simulink model "JABS_AutoSave_20200707_1036"  (R2018b)
settings: Solver=FixedStepAuto  StartTime=0.0  StopTime=10.0  FixedStep=0.01  RelTol=1e-3
(part 2 of 2)

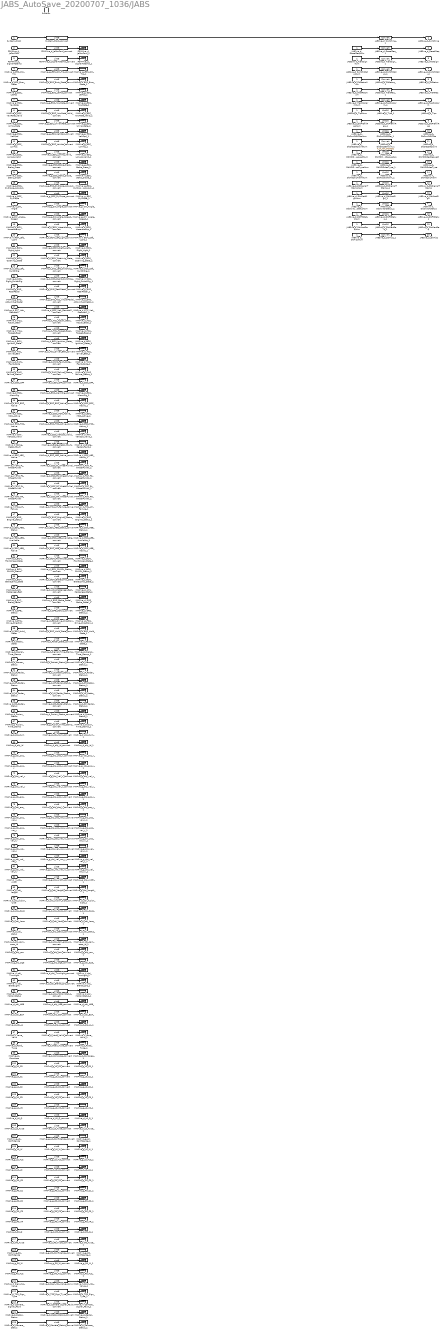
== system JABS_AutoSave_20200707_1036/JABS ==
  System_Clock : Inport  OutDataTypeStr=UInt16
  FDMMve_d_JaFcnConf : Inport  Port=2  OutDataTypeStr=UInt16
  FDMMve_d_SignalTStamp : Inport  Port=3  OutDataTypeStr=UInt16
  IMAPve_g_EPS_SW_Trq : Inport  Port=4  OutDataTypeStr=T_M_Nm_Float32
  IMAPve_d_EPS_Error_State : Inport  Port=5  OutDataTypeStr=UInt16
  IMAPve_g_ESC_LatAcc : Inport  Port=6  OutDataTypeStr=T_M_Nm_Float32
  IMAPve_g_ESC_YawRate : Inport  Port=7  OutDataTypeStr=T_M_Nm_Float32
  IMAPve_d_ESC_YawRate_Valid : Inport  Port=8  OutDataTypeStr=UInt16
  IMAPve_g_ESC_UnYawRate : Inport  Port=9  OutDataTypeStr=T_M_Nm_Float32
  IMAPve_g_ESC_VehSpd : Inport  Port=10  OutDataTypeStr=T_M_Nm_Float32
  IMAPve_g_ESC_LonAcc : Inport  Port=11  OutDataTypeStr=T_M_Nm_Float32
  IMAPve_d_ESC_LonAcc_Valid : Inport  Port=12  OutDataTypeStr=UInt16
  IMAPve_g_ESC_Brake_Press : Inport  Port=13  OutDataTypeStr=T_M_Nm_Float32
  IMAPve_g_ESC_Static_Slope : Inport  Port=14  OutDataTypeStr=T_M_Nm_Float32
  IMAPve_g_ESC_DySlope_Accuracy : Inport  Port=15  OutDataTypeStr=T_M_Nm_Float32
  IMAPve_g_ESC_DySlope : Inport  Port=16  OutDataTypeStr=T_M_Nm_Float32
  IMAPve_g_SW_Angle : Inport  Port=17  OutDataTypeStr=T_M_Nm_Float32
  IMAPve_g_SW_Angle_Speed : Inport  Port=18  OutDataTypeStr=T_M_Nm_Float32
  IMAPve_d_BCM_HazardLamp : Inport  Port=19  OutDataTypeStr=UInt16
  IMAPve_d_BCM_Left_Light : Inport  Port=20  OutDataTypeStr=UInt16
  IMAPve_d_BCM_Right_Light : Inport  Port=21  OutDataTypeStr=UInt16
  IMAPve_d_BCM_Opening_State : Inport  Port=22  OutDataTypeStr=UInt16
  IMAPve_d_SCC_Left_SwitchSig : Inport  Port=23  OutDataTypeStr=UInt16
  IMAPve_d_SCC_Right_SwitchSig : Inport  Port=24  OutDataTypeStr=UInt16
  IMAPve_g_EMS_RealPedal : Inport  Port=25  OutDataTypeStr=T_M_Nm_Float32
  IMAPve_g_EMS_ACC_VirtualPedal : Inport  Port=26  OutDataTypeStr=T_M_Nm_Float32
  IMAPve_d_ESC_Veh_Standstill : Inport  Port=27  OutDataTypeStr=UInt16
  IMAPve_d_TCU_Actual_Gear : Inport  Port=28  OutDataTypeStr=UInt16
  IMAPve_d_TCU_Target_Gear : Inport  Port=29  OutDataTypeStr=UInt16
  IMAPve_d_BCM_Ignition_State : Inport  Port=30  OutDataTypeStr=UInt16
  IMAPve_d_ACU_Driver_Belt : Inport  Port=31  OutDataTypeStr=UInt16
  IMAPve_d_SWS_Fault_Code : Inport  Port=32  OutDataTypeStr=UInt16
  IMAPve_d_SWS_Failure_Status : Inport  Port=33  OutDataTypeStr=UInt16
  IMAPve_d_ESC_OFF : Inport  Port=34  OutDataTypeStr=UInt16
  IMAPve_d_ESC_AlarmSig : Inport  Port=35  OutDataTypeStr=UInt16
  IMAPve_d_ESC_ESC_Active : Inport  Port=36  OutDataTypeStr=UInt16
  IMAPve_d_ESC_MSR_Active : Inport  Port=37  OutDataTypeStr=UInt16
  IMAPve_d_ESC_TCS_Active : Inport  Port=38  OutDataTypeStr=UInt16
  IMAPve_d_ESC_VehSpd_Valid : Inport  Port=39  OutDataTypeStr=UInt16
  IMAPve_d_Brake_Pedal_Fault : Inport  Port=40  OutDataTypeStr=UInt16
  IMAPve_d_ESC_ABS_Active : Inport  Port=41  OutDataTypeStr=UInt16
  IMAPve_d_ESC_FL_WheelPulVal : Inport  Port=42  OutDataTypeStr=UInt16
  IMAPve_d_ESC_FR_WheelPulVal : Inport  Port=43  OutDataTypeStr=UInt16
  IMAPve_d_ESC_RL_WheelPulVal : Inport  Port=44  OutDataTypeStr=UInt16
  IMAPve_d_ESC_RR_WheelPulVal : Inport  Port=45  OutDataTypeStr=UInt16
  IMAPve_d_TCU_AT_Failure : Inport  Port=46  OutDataTypeStr=UInt16
  IMAPve_d_EMS_Engine_Status : Inport  Port=47  OutDataTypeStr=UInt16
  IMAPve_d_ESC_AEB_Status : Inport  Port=48  OutDataTypeStr=UInt16
  IMAPve_d_ESC_AEB_Available : Inport  Port=49  OutDataTypeStr=UInt16
  IMAPve_d_ESC_AEB_Active : Inport  Port=50  OutDataTypeStr=UInt16
  IMAPve_d_BCM_FrontWiper_State : Inport  Port=51  OutDataTypeStr=UInt16
  IMAPve_d_BCM_CHMSL_Status : Inport  Port=52  OutDataTypeStr=UInt16
  IMAPve_d_BCM_BrakeLamp_State : Inport  Port=53  OutDataTypeStr=UInt16
  IMAPve_d_ACU_Passenger_Belt : Inport  Port=54  OutDataTypeStr=UInt16
  IMAPve_d_EMS_Brake_Pedal : Inport  Port=55  OutDataTypeStr=UInt16
  IMAPve_d_EPB_Status : Inport  Port=56  OutDataTypeStr=UInt16
  IMAPve_d_ESC_Drive_Direction : Inport  Port=57  OutDataTypeStr=UInt16
  IMAPve_d_ESC_Hold_State : Inport  Port=58  OutDataTypeStr=UInt16
  IMAPve_d_Radar_State : Inport  Port=59  OutDataTypeStr=UInt16
  IMAPve_d_Signal_Time_Stamp : Inport  Port=60  OutDataTypeStr=UInt16
  IMAPve_d_Sensor_Status : Inport  Port=61  OutDataTypeStr=UInt16
  IMAPve_d_LF_Radar_Status : Inport  Port=62  OutDataTypeStr=UInt16
  IMAPve_d_RF_Radar_Status : Inport  Port=63  OutDataTypeStr=UInt16
  IMAPve_d_LR_Radar_Status : Inport  Port=64  OutDataTypeStr=UInt16
  IMAPve_d_RR_Radar_Status : Inport  Port=65  OutDataTypeStr=UInt16
  IMAPve_d_Fusion_Status : Inport  Port=66  OutDataTypeStr=UInt16
  IMAPve_g_Fusion_Time_Stamp : Inport  Port=67  OutDataTypeStr=T_M_Nm_Float32
  IMAPve_d_obj_Num : Inport  Port=68  OutDataTypeStr=UInt16
  IMAPva_d_obj_id : Inport  Port=69  OutDataTypeStr=UInt16  PortDimensions=40
  IMAPva_g_obj_pos_x : Inport  Port=70  OutDataTypeStr=T_M_Nm_Float32  PortDimensions=40
  IMAPva_g_obj_pos_y : Inport  Port=71  OutDataTypeStr=T_M_Nm_Float32  PortDimensions=40
  IMAPva_g_obj_vel_x : Inport  Port=72  OutDataTypeStr=T_M_Nm_Float32  PortDimensions=40
  IMAPva_g_obj_vel_y : Inport  Port=73  OutDataTypeStr=T_M_Nm_Float32  PortDimensions=40
  IMAPva_g_obj_acc_x : Inport  Port=74  OutDataTypeStr=T_M_Nm_Float32  PortDimensions=40
  IMAPva_g_obj_acc_y : Inport  Port=75  OutDataTypeStr=T_M_Nm_Float32  PortDimensions=40
  IMAPva_g_obj_pos_var_x : Inport  Port=76  OutDataTypeStr=T_M_Nm_Float32  PortDimensions=40
  IMAPva_g_obj_pos_var_y : Inport  Port=77  OutDataTypeStr=T_M_Nm_Float32  PortDimensions=40
  IMAPva_g_obj_pos_var_xy : Inport  Port=78  OutDataTypeStr=T_M_Nm_Float32  PortDimensions=40
  IMAPva_g_obj_vel_var_x : Inport  Port=79  OutDataTypeStr=T_M_Nm_Float32  PortDimensions=40
  IMAPva_g_obj_vel_var_y : Inport  Port=80  OutDataTypeStr=T_M_Nm_Float32  PortDimensions=40
  IMAPva_g_obj_vel_var_xy : Inport  Port=81  OutDataTypeStr=T_M_Nm_Float32  PortDimensions=40
  IMAPva_g_obj_width : Inport  Port=82  OutDataTypeStr=T_M_Nm_Float32  PortDimensions=40
  IMAPva_g_obj_length : Inport  Port=83  OutDataTypeStr=T_M_Nm_Float32  PortDimensions=40
  IMAPva_d_obj_fusion_type : Inport  Port=84  OutDataTypeStr=UInt16  PortDimensions=40
  IMAPva_d_obj_class : Inport  Port=85  OutDataTypeStr=UInt16  PortDimensions=40
  IMAPva_d_obj_lane : Inport  Port=86  OutDataTypeStr=UInt16  PortDimensions=40
  IMAPva_d_obj_status : Inport  Port=87  OutDataTypeStr=UInt16  PortDimensions=40
  IMAPva_d_obj_cam_asso_id : Inport  Port=88  OutDataTypeStr=UInt16  PortDimensions=40
  IMAPva_g_obj_con : Inport  Port=89  OutDataTypeStr=T_M_Nm_Float32  PortDimensions=40
  IMAPva_g_obj_age : Inport  Port=90  OutDataTypeStr=T_M_Nm_Float32  PortDimensions=40
  IMAPva_d_obj_TurnLight : Inport  Port=91  OutDataTypeStr=UInt16  PortDimensions=40
  IMAPva_d_obj_BrakeLight : Inport  Port=92  OutDataTypeStr=UInt16  PortDimensions=40
  IMAPva_d_obj_MotionStatus : Inport  Port=93  OutDataTypeStr=UInt16  PortDimensions=40
  IMAPva_d_obj_AEB : Inport  Port=94  OutDataTypeStr=UInt16  PortDimensions=40
  IMAPva_d_obj_ESA : Inport  Port=95  OutDataTypeStr=UInt16  PortDimensions=40
  IMAPva_d_obj_JA : Inport  Port=96  OutDataTypeStr=UInt16  PortDimensions=40
  IMAPve_d_Lane_Valid : Inport  Port=97  OutDataTypeStr=UInt16
  IMAPve_d_Road_Type : Inport  Port=98  OutDataTypeStr=UInt16
  IMAPve_d_ConsArea : Inport  Port=99  OutDataTypeStr=UInt16
  IMAPve_g_L0_C0 : Inport  Port=100  OutDataTypeStr=T_M_Nm_Float32
  IMAPve_g_L0_C1 : Inport  Port=101  OutDataTypeStr=T_M_Nm_Float32
  IMAPve_g_L0_C2 : Inport  Port=102  OutDataTypeStr=T_M_Nm_Float32
  IMAPve_g_L0_C3 : Inport  Port=103  OutDataTypeStr=T_M_Nm_Float32
  IMAPve_g_L0_VR : Inport  Port=104  OutDataTypeStr=T_M_Nm_Float32
  IMAPve_d_L0_Q : Inport  Port=105  OutDataTypeStr=UInt16
  IMAPve_d_L0_Type : Inport  Port=106  OutDataTypeStr=UInt16
  IMAPve_g_L0_Confidence : Inport  Port=107  OutDataTypeStr=T_M_Nm_Float32
  IMAPve_g_L0_W : Inport  Port=108  OutDataTypeStr=T_M_Nm_Float32
  IMAPve_g_L0_TLC : Inport  Port=109  OutDataTypeStr=T_M_Nm_Float32
  IMAPve_d_L0_LC : Inport  Port=110  OutDataTypeStr=UInt16
  IMAPve_g_R0_C0 : Inport  Port=111  OutDataTypeStr=T_M_Nm_Float32
  IMAPve_g_R0_C1 : Inport  Port=112  OutDataTypeStr=T_M_Nm_Float32
  IMAPve_g_R0_C2 : Inport  Port=113  OutDataTypeStr=T_M_Nm_Float32
  IMAPve_g_R0_C3 : Inport  Port=114  OutDataTypeStr=T_M_Nm_Float32
  IMAPve_g_R0_VR : Inport  Port=115  OutDataTypeStr=T_M_Nm_Float32
  IMAPve_d_R0_Q : Inport  Port=116  OutDataTypeStr=UInt16
  IMAPve_d_R0_Type : Inport  Port=117  OutDataTypeStr=UInt16
  IMAPve_g_R0_Confidence : Inport  Port=118  OutDataTypeStr=T_M_Nm_Float32
  IMAPve_g_R0_W : Inport  Port=119  OutDataTypeStr=T_M_Nm_Float32
  IMAPve_g_R0_TLC : Inport  Port=120  OutDataTypeStr=T_M_Nm_Float32
  IMAPve_d_Sign_ISA_Value : Inport  Port=121  OutDataTypeStr=UInt16
  IMAPve_d_TSR_Sign_Type : Inport  Port=122  OutDataTypeStr=UInt16
  IMAPve_d_Camera_Signal_Fault : Inport  Port=123  OutDataTypeStr=UInt16
  IMAPve_d_Radar_Status : Inport  Port=124  OutDataTypeStr=UInt16
  IMAPve_d_Camera_Status : Inport  Port=125  OutDataTypeStr=UInt16
  function : TriggerPort  TriggerType=function-call  VariantControl=Variant  SampleTimeType=periodic  SampleTime=-1
  FDMMve_d_JaFcnConf_1 : Terminator
  FDMMve_d_JaFcnConf_convert : DataTypeConversion  OutDataTypeStr=uint8
  FDMMve_d_SignalTStamp_1 : Terminator
  FDMMve_d_SignalTStamp_convert : DataTypeConversion  OutDataTypeStr=uint8
  IMAPva_d_obj_AEB_1 : Terminator
  IMAPva_d_obj_AEB_convert : DataTypeConversion  OutDataTypeStr=uint8
  IMAPva_d_obj_BrakeLight_1 : Terminator
  IMAPva_d_obj_BrakeLight_convert : DataTypeConversion  OutDataTypeStr=uint8
  IMAPva_d_obj_ESA_1 : Terminator
  IMAPva_d_obj_ESA_convert : DataTypeConversion  OutDataTypeStr=uint8
  IMAPva_d_obj_JA_1 : Terminator
  IMAPva_d_obj_JA_convert : DataTypeConversion  OutDataTypeStr=uint8
  IMAPva_d_obj_MotionStatus_1 : Terminator
  IMAPva_d_obj_MotionStatus_convert : DataTypeConversion  OutDataTypeStr=uint8
  IMAPva_d_obj_TurnLight_1 : Terminator
  IMAPva_d_obj_TurnLight_convert : DataTypeConversion  OutDataTypeStr=uint8
  IMAPva_d_obj_cam_asso_id_1 : Terminator
  IMAPva_d_obj_cam_asso_id_convert : DataTypeConversion  OutDataTypeStr=uint8
  IMAPva_d_obj_class_1 : Terminator
  IMAPva_d_obj_class_convert : DataTypeConversion  OutDataTypeStr=uint8
  IMAPva_d_obj_fusion_type_1 : Terminator
  IMAPva_d_obj_fusion_type_convert : DataTypeConversion  OutDataTypeStr=uint8
  IMAPva_d_obj_id_1 : Terminator
  IMAPva_d_obj_id_convert : DataTypeConversion  OutDataTypeStr=uint8
  IMAPva_d_obj_lane_1 : Terminator
  IMAPva_d_obj_lane_convert : DataTypeConversion  OutDataTypeStr=uint8
  IMAPva_d_obj_status_1 : Terminator
  IMAPva_d_obj_status_convert : DataTypeConversion  OutDataTypeStr=uint8
  IMAPva_g_obj_acc_x_1 : Terminator
  IMAPva_g_obj_acc_x_convert : DataTypeConversion  OutDataTypeStr=uint8
  IMAPva_g_obj_acc_y_1 : Terminator
  IMAPva_g_obj_acc_y_convert : DataTypeConversion  OutDataTypeStr=uint8
  IMAPva_g_obj_age_1 : Terminator
  IMAPva_g_obj_age_convert : DataTypeConversion  OutDataTypeStr=uint8
  IMAPva_g_obj_con_1 : Terminator
  IMAPva_g_obj_con_convert : DataTypeConversion  OutDataTypeStr=uint8
  IMAPva_g_obj_length_1 : Terminator
  IMAPva_g_obj_length_convert : DataTypeConversion  OutDataTypeStr=uint8
  IMAPva_g_obj_pos_var_x_1 : Terminator
  IMAPva_g_obj_pos_var_x_convert : DataTypeConversion  OutDataTypeStr=uint8
  IMAPva_g_obj_pos_var_xy_1 : Terminator
  IMAPva_g_obj_pos_var_xy_convert : DataTypeConversion  OutDataTypeStr=uint8
  IMAPva_g_obj_pos_var_y_1 : Terminator
  IMAPva_g_obj_pos_var_y_convert : DataTypeConversion  OutDataTypeStr=uint8
  IMAPva_g_obj_pos_x_1 : Terminator
  IMAPva_g_obj_pos_x_convert : DataTypeConversion  OutDataTypeStr=uint8
  IMAPva_g_obj_pos_y_1 : Terminator
  IMAPva_g_obj_pos_y_convert : DataTypeConversion  OutDataTypeStr=uint8
  IMAPva_g_obj_vel_var_x_1 : Terminator
  IMAPva_g_obj_vel_var_x_convert : DataTypeConversion  OutDataTypeStr=uint8
  IMAPva_g_obj_vel_var_xy_1 : Terminator
  IMAPva_g_obj_vel_var_xy_convert : DataTypeConversion  OutDataTypeStr=uint8
  IMAPva_g_obj_vel_var_y_1 : Terminator
  IMAPva_g_obj_vel_var_y_convert : DataTypeConversion  OutDataTypeStr=uint8
  IMAPva_g_obj_vel_x_1 : Terminator
  IMAPva_g_obj_vel_x_convert : DataTypeConversion  OutDataTypeStr=uint8
  IMAPva_g_obj_vel_y_1 : Terminator
  IMAPva_g_obj_vel_y_convert : DataTypeConversion  OutDataTypeStr=uint8
  IMAPva_g_obj_width_1 : Terminator
  IMAPva_g_obj_width_convert : DataTypeConversion  OutDataTypeStr=uint8
  IMAPve_d_ACU_Driver_Belt_1 : Terminator
  IMAPve_d_ACU_Driver_Belt_convert : DataTypeConversion  OutDataTypeStr=uint8
  IMAPve_d_ACU_Passenger_Belt_1 : Terminator
  IMAPve_d_ACU_Passenger_Belt_convert : DataTypeConversion  OutDataTypeStr=uint8
  IMAPve_d_BCM_BrakeLamp_State_1 : Terminator
  IMAPve_d_BCM_BrakeLamp_State_convert : DataTypeConversion  OutDataTypeStr=uint8
  IMAPve_d_BCM_CHMSL_Status_1 : Terminator
  IMAPve_d_BCM_CHMSL_Status_convert : DataTypeConversion  OutDataTypeStr=uint8
  IMAPve_d_BCM_FrontWiper_State_1 : Terminator
  IMAPve_d_BCM_FrontWiper_State_convert : DataTypeConversion  OutDataTypeStr=uint8
  IMAPve_d_BCM_HazardLamp_1 : Terminator
  IMAPve_d_BCM_HazardLamp_convert : DataTypeConversion  OutDataTypeStr=uint8
  IMAPve_d_BCM_Ignition_State_1 : Terminator
  IMAPve_d_BCM_Ignition_State_convert : DataTypeConversion  OutDataTypeStr=uint8
  IMAPve_d_BCM_Left_Light_1 : Terminator
  IMAPve_d_BCM_Left_Light_convert : DataTypeConversion  OutDataTypeStr=uint8
  IMAPve_d_BCM_Opening_State_1 : Terminator
  IMAPve_d_BCM_Opening_State_convert : DataTypeConversion  OutDataTypeStr=uint8
  IMAPve_d_BCM_Right_Light_1 : Terminator
  IMAPve_d_BCM_Right_Light_convert : DataTypeConversion  OutDataTypeStr=uint8
  IMAPve_d_Brake_Pedal_Fault_1 : Terminator
  IMAPve_d_Brake_Pedal_Fault_convert : DataTypeConversion  OutDataTypeStr=uint8
  IMAPve_d_Camera_Signal_Fault_1 : Terminator
  IMAPve_d_Camera_Signal_Fault_convert : DataTypeConversion  OutDataTypeStr=uint8
  IMAPve_d_Camera_Status_1 : Terminator
  IMAPve_d_Camera_Status_convert : DataTypeConversion  OutDataTypeStr=uint8
  IMAPve_d_ConsArea_1 : Terminator
  IMAPve_d_ConsArea_convert : DataTypeConversion  OutDataTypeStr=uint8
  IMAPve_d_EMS_Brake_Pedal_1 : Terminator
  IMAPve_d_EMS_Brake_Pedal_convert : DataTypeConversion  OutDataTypeStr=uint8
  IMAPve_d_EMS_Engine_Status_1 : Terminator
  IMAPve_d_EMS_Engine_Status_convert : DataTypeConversion  OutDataTypeStr=uint8
  IMAPve_d_EPB_Status_1 : Terminator
  IMAPve_d_EPB_Status_convert : DataTypeConversion  OutDataTypeStr=uint8
  IMAPve_d_EPS_Error_State_1 : Terminator
  IMAPve_d_EPS_Error_State_convert : DataTypeConversion  OutDataTypeStr=uint8
  IMAPve_d_ESC_ABS_Active_1 : Terminator
  IMAPve_d_ESC_ABS_Active_convert : DataTypeConversion  OutDataTypeStr=uint8
  IMAPve_d_ESC_AEB_Active_1 : Terminator
  IMAPve_d_ESC_AEB_Active_convert : DataTypeConversion  OutDataTypeStr=uint8
  IMAPve_d_ESC_AEB_Available_1 : Terminator
  IMAPve_d_ESC_AEB_Available_convert : DataTypeConversion  OutDataTypeStr=uint8
  IMAPve_d_ESC_AEB_Status_1 : Terminator
  IMAPve_d_ESC_AEB_Status_convert : DataTypeConversion  OutDataTypeStr=uint8
  IMAPve_d_ESC_AlarmSig_1 : Terminator
  IMAPve_d_ESC_AlarmSig_convert : DataTypeConversion  OutDataTypeStr=uint8
  IMAPve_d_ESC_Drive_Direction_1 : Terminator
  IMAPve_d_ESC_Drive_Direction_convert : DataTypeConversion  OutDataTypeStr=uint8
  IMAPve_d_ESC_ESC_Active_1 : Terminator
  IMAPve_d_ESC_ESC_Active_convert : DataTypeConversion  OutDataTypeStr=uint8
  IMAPve_d_ESC_FL_WheelPulVal_1 : Terminator
  IMAPve_d_ESC_FL_WheelPulVal_convert : DataTypeConversion  OutDataTypeStr=uint8
  IMAPve_d_ESC_FR_WheelPulVal_1 : Terminator
  IMAPve_d_ESC_FR_WheelPulVal_convert : DataTypeConversion  OutDataTypeStr=uint8
  IMAPve_d_ESC_Hold_State_1 : Terminator
  IMAPve_d_ESC_Hold_State_convert : DataTypeConversion  OutDataTypeStr=uint8
  IMAPve_d_ESC_LonAcc_Valid_1 : Terminator
  IMAPve_d_ESC_LonAcc_Valid_convert : DataTypeConversion  OutDataTypeStr=uint8
  IMAPve_d_ESC_MSR_Active_1 : Terminator
  IMAPve_d_ESC_MSR_Active_convert : DataTypeConversion  OutDataTypeStr=uint8
  IMAPve_d_ESC_OFF_1 : Terminator
  IMAPve_d_ESC_OFF_convert : DataTypeConversion  OutDataTypeStr=uint8
  IMAPve_d_ESC_RL_WheelPulVal_1 : Terminator
  IMAPve_d_ESC_RL_WheelPulVal_convert : DataTypeConversion  OutDataTypeStr=uint8
  IMAPve_d_ESC_RR_WheelPulVal_1 : Terminator
  IMAPve_d_ESC_RR_WheelPulVal_convert : DataTypeConversion  OutDataTypeStr=uint8
  IMAPve_d_ESC_TCS_Active_1 : Terminator
  IMAPve_d_ESC_TCS_Active_convert : DataTypeConversion  OutDataTypeStr=uint8
  IMAPve_d_ESC_VehSpd_Valid_1 : Terminator
  IMAPve_d_ESC_VehSpd_Valid_convert : DataTypeConversion  OutDataTypeStr=uint8
  IMAPve_d_ESC_Veh_Standstill_1 : Terminator
  IMAPve_d_ESC_Veh_Standstill_convert : DataTypeConversion  OutDataTypeStr=uint8
  IMAPve_d_ESC_YawRate_Valid_1 : Terminator
  IMAPve_d_ESC_YawRate_Valid_convert : DataTypeConversion  OutDataTypeStr=uint8
  IMAPve_d_Fusion_Status_1 : Terminator
  IMAPve_d_Fusion_Status_convert : DataTypeConversion  OutDataTypeStr=uint8
  IMAPve_d_L0_LC_1 : Terminator
  IMAPve_d_L0_LC_convert : DataTypeConversion  OutDataTypeStr=uint8
  IMAPve_d_L0_Q_1 : Terminator
  IMAPve_d_L0_Q_convert : DataTypeConversion  OutDataTypeStr=uint8
  IMAPve_d_L0_Type_1 : Terminator
  IMAPve_d_L0_Type_convert : DataTypeConversion  OutDataTypeStr=uint8
  IMAPve_d_LF_Radar_Status_1 : Terminator
  IMAPve_d_LF_Radar_Status_convert : DataTypeConversion  OutDataTypeStr=uint8
  IMAPve_d_LR_Radar_Status_1 : Terminator
  IMAPve_d_LR_Radar_Status_convert : DataTypeConversion  OutDataTypeStr=uint8
  IMAPve_d_Lane_Valid_1 : Terminator
  IMAPve_d_Lane_Valid_convert : DataTypeConversion  OutDataTypeStr=uint8
  IMAPve_d_R0_Q_1 : Terminator
  IMAPve_d_R0_Q_convert : DataTypeConversion  OutDataTypeStr=uint8
  IMAPve_d_R0_Type_1 : Terminator
  IMAPve_d_R0_Type_convert : DataTypeConversion  OutDataTypeStr=uint8
  IMAPve_d_RF_Radar_Status_1 : Terminator
  IMAPve_d_RF_Radar_Status_convert : DataTypeConversion  OutDataTypeStr=uint8
  IMAPve_d_RR_Radar_Status_1 : Terminator
  IMAPve_d_RR_Radar_Status_convert : DataTypeConversion  OutDataTypeStr=uint8
  IMAPve_d_Radar_State_1 : Terminator
  IMAPve_d_Radar_State_convert : DataTypeConversion  OutDataTypeStr=uint8
  IMAPve_d_Radar_Status_1 : Terminator
  IMAPve_d_Radar_Status_convert : DataTypeConversion  OutDataTypeStr=uint8
  IMAPve_d_Road_Type_1 : Terminator
  IMAPve_d_Road_Type_convert : DataTypeConversion  OutDataTypeStr=uint8
  IMAPve_d_SCC_Left_SwitchSig_1 : Terminator
  IMAPve_d_SCC_Left_SwitchSig_convert : DataTypeConversion  OutDataTypeStr=uint8
  IMAPve_d_SCC_Right_SwitchSig_1 : Terminator
  IMAPve_d_SCC_Right_SwitchSig_convert : DataTypeConversion  OutDataTypeStr=uint8
  IMAPve_d_SWS_Failure_Status_1 : Terminator
  IMAPve_d_SWS_Failure_Status_convert : DataTypeConversion  OutDataTypeStr=uint8
  IMAPve_d_SWS_Fault_Code_1 : Terminator
  IMAPve_d_SWS_Fault_Code_convert : DataTypeConversion  OutDataTypeStr=uint8
  IMAPve_d_Sensor_Status_1 : Terminator
  IMAPve_d_Sensor_Status_convert : DataTypeConversion  OutDataTypeStr=uint8
  IMAPve_d_Sign_ISA_Value_1 : Terminator
  IMAPve_d_Sign_ISA_Value_convert : DataTypeConversion  OutDataTypeStr=uint8
  IMAPve_d_Signal_Time_Stamp_1 : Terminator
  IMAPve_d_Signal_Time_Stamp_convert : DataTypeConversion  OutDataTypeStr=uint8
  IMAPve_d_TCU_AT_Failure_1 : Terminator
  IMAPve_d_TCU_AT_Failure_convert : DataTypeConversion  OutDataTypeStr=uint8
  IMAPve_d_TCU_Actual_Gear_1 : Terminator
  IMAPve_d_TCU_Actual_Gear_convert : DataTypeConversion  OutDataTypeStr=uint8
  IMAPve_d_TCU_Target_Gear_1 : Terminator
  IMAPve_d_TCU_Target_Gear_convert : DataTypeConversion  OutDataTypeStr=uint8
  IMAPve_d_TSR_Sign_Type_1 : Terminator
  IMAPve_d_TSR_Sign_Type_convert : DataTypeConversion  OutDataTypeStr=uint8
  IMAPve_d_obj_Num_1 : Terminator
  IMAPve_d_obj_Num_convert : DataTypeConversion  OutDataTypeStr=uint8
  IMAPve_g_EMS_ACC_VirtualPedal_1 : Terminator
  IMAPve_g_EMS_ACC_VirtualPedal_convert : DataTypeConversion  OutDataTypeStr=uint8
  IMAPve_g_EMS_RealPedal_1 : Terminator
  IMAPve_g_EMS_RealPedal_convert : DataTypeConversion  OutDataTypeStr=uint8
  IMAPve_g_EPS_SW_Trq_1 : Terminator
  IMAPve_g_EPS_SW_Trq_convert : DataTypeConversion  OutDataTypeStr=uint8
  IMAPve_g_ESC_Brake_Press_1 : Terminator
  IMAPve_g_ESC_Brake_Press_convert : DataTypeConversion  OutDataTypeStr=uint8
  IMAPve_g_ESC_DySlope_1 : Terminator
  IMAPve_g_ESC_DySlope_Accuracy_1 : Terminator
  IMAPve_g_ESC_DySlope_Accuracy_convert : DataTypeConversion  OutDataTypeStr=uint8
  IMAPve_g_ESC_DySlope_convert : DataTypeConversion  OutDataTypeStr=uint8
  IMAPve_g_ESC_LatAcc_1 : Terminator
  IMAPve_g_ESC_LatAcc_convert : DataTypeConversion  OutDataTypeStr=uint8
  IMAPve_g_ESC_LonAcc_1 : Terminator
  IMAPve_g_ESC_LonAcc_convert : DataTypeConversion  OutDataTypeStr=uint8
  IMAPve_g_ESC_Static_Slope_1 : Terminator
  IMAPve_g_ESC_Static_Slope_convert : DataTypeConversion  OutDataTypeStr=uint8
  IMAPve_g_ESC_UnYawRate_1 : Terminator
  IMAPve_g_ESC_UnYawRate_convert : DataTypeConversion  OutDataTypeStr=uint8
  IMAPve_g_ESC_VehSpd_1 : Terminator
  IMAPve_g_ESC_VehSpd_convert : DataTypeConversion  OutDataTypeStr=uint8
  IMAPve_g_ESC_YawRate_1 : Terminator
  IMAPve_g_ESC_YawRate_convert : DataTypeConversion  OutDataTypeStr=uint8
  IMAPve_g_Fusion_Time_Stamp_1 : Terminator
  IMAPve_g_Fusion_Time_Stamp_convert : DataTypeConversion  OutDataTypeStr=uint8
  IMAPve_g_L0_C0_1 : Terminator
  IMAPve_g_L0_C0_convert : DataTypeConversion  OutDataTypeStr=uint8
  IMAPve_g_L0_C1_1 : Terminator
  IMAPve_g_L0_C1_convert : DataTypeConversion  OutDataTypeStr=uint8
  IMAPve_g_L0_C2_1 : Terminator
  IMAPve_g_L0_C2_convert : DataTypeConversion  OutDataTypeStr=uint8
  IMAPve_g_L0_C3_1 : Terminator
  IMAPve_g_L0_C3_convert : DataTypeConversion  OutDataTypeStr=uint8
  IMAPve_g_L0_Confidence_1 : Terminator
  IMAPve_g_L0_Confidence_convert : DataTypeConversion  OutDataTypeStr=uint8
  IMAPve_g_L0_TLC_1 : Terminator
  IMAPve_g_L0_TLC_convert : DataTypeConversion  OutDataTypeStr=uint8
  IMAPve_g_L0_VR_1 : Terminator
  IMAPve_g_L0_VR_convert : DataTypeConversion  OutDataTypeStr=uint8
  IMAPve_g_L0_W_1 : Terminator
  IMAPve_g_L0_W_convert : DataTypeConversion  OutDataTypeStr=uint8
  IMAPve_g_R0_C0_1 : Terminator
  IMAPve_g_R0_C0_convert : DataTypeConversion  OutDataTypeStr=uint8
  IMAPve_g_R0_C1_1 : Terminator
  IMAPve_g_R0_C1_convert : DataTypeConversion  OutDataTypeStr=uint8
  IMAPve_g_R0_C2_1 : Terminator
  IMAPve_g_R0_C2_convert : DataTypeConversion  OutDataTypeStr=uint8
  IMAPve_g_R0_C3_1 : Terminator
  IMAPve_g_R0_C3_convert : DataTypeConversion  OutDataTypeStr=uint8
  IMAPve_g_R0_Confidence_1 : Terminator
  IMAPve_g_R0_Confidence_convert : DataTypeConversion  OutDataTypeStr=uint8
  IMAPve_g_R0_TLC_1 : Terminator
  IMAPve_g_R0_TLC_convert : DataTypeConversion  OutDataTypeStr=uint8
  IMAPve_g_R0_VR_1 : Terminator
  IMAPve_g_R0_VR_convert : DataTypeConversion  OutDataTypeStr=uint8
  IMAPve_g_R0_W_1 : Terminator
  IMAPve_g_R0_W_convert : DataTypeConversion  OutDataTypeStr=uint8
  IMAPve_g_SW_Angle_1 : Terminator
  IMAPve_g_SW_Angle_Speed_1 : Terminator
  IMAPve_g_SW_Angle_Speed_convert : DataTypeConversion  OutDataTypeStr=uint8
  IMAPve_g_SW_Angle_convert : DataTypeConversion  OutDataTypeStr=uint8
  JABSve_d_AlertReqNum : Constant  OutDataTypeStr=uint8
  JABSve_d_AlertReq_1 : DataTypeConversion
  JABSve_d_AlertSignNum : Constant  OutDataTypeStr=uint8  SampleTime=-1
  JABSve_d_AlertSign_1 : DataTypeConversion
  JABSve_d_DbAlertReqNum : Constant  OutDataTypeStr=uint8
  JABSve_d_DbAlertReq_1 : DataTypeConversion  OutDataTypeStr=UInt16
  JABSve_d_DbAlertSignNum : Constant  OutDataTypeStr=uint8
  JABSve_d_DbAlertSign_1 : DataTypeConversion  OutDataTypeStr=UInt16
  JABSve_d_DbDecSetpointNum : Constant  OutDataTypeStr=uint8
  JABSve_d_DbDecSetpoint_1 : DataTypeConversion  OutDataTypeStr=T_M_Nm_Float32
  JABSve_d_DbFltStatusNum : Constant  OutDataTypeStr=uint8
  JABSve_d_DbFltStatus_1 : DataTypeConversion  OutDataTypeStr=UInt16
  JABSve_d_DbFunFARCStaNum : Constant  OutDataTypeStr=uint8
  JABSve_d_DbFunFARCSta_1 : DataTypeConversion  OutDataTypeStr=UInt16
  JABSve_d_DbHapticAlarmNum : Constant  OutDataTypeStr=uint8
  JABSve_d_DbHapticAlarm_1 : DataTypeConversion  OutDataTypeStr=UInt16
  JABSve_d_DbMDDdecRequestNum : Constant  OutDataTypeStr=uint8
  JABSve_d_DbMDDdecRequest_1 : DataTypeConversion  OutDataTypeStr=UInt16
  JABSve_d_DbMDDdecTypeNum : Constant  OutDataTypeStr=uint8
  JABSve_d_DbMDDdecType_1 : DataTypeConversion  OutDataTypeStr=UInt16
  JABSve_d_DbPrefillReqNum : Constant  OutDataTypeStr=uint8
  JABSve_d_DbPrefillReq_1 : DataTypeConversion  OutDataTypeStr=UInt16
  JABSve_d_DbSignalTStampNum : Constant  OutDataTypeStr=uint8
  JABSve_d_DbSignalTStamp_1 : DataTypeConversion  OutDataTypeStr=UInt16
  JABSve_d_DbSwitchStatusNum : Constant  OutDataTypeStr=uint8
  JABSve_d_DbSwitchStatus_1 : DataTypeConversion  OutDataTypeStr=UInt16
  JABSve_d_DbTipsNum : Constant  OutDataTypeStr=uint8
  JABSve_d_DbTips_1 : DataTypeConversion
  JABSve_d_DecelReqNum : Constant  OutDataTypeStr=uint8
  JABSve_d_DecelReq_1 : DataTypeConversion
  JABSve_d_FltStatusNum : Constant  OutDataTypeStr=uint8
  JABSve_d_FltStatus_1 : DataTypeConversion
  JABSve_d_HapticAlarmNum : Constant  OutDataTypeStr=uint8
  JABSve_d_HapticAlarm_1 : DataTypeConversion
  JABSve_d_SwitchStatusNum : Constant  OutDataTypeStr=uint8  SampleTime=-1
  JABSve_d_SwitchStatus_1 : DataTypeConversion
  JABSve_d_Switching_1 : DataTypeConversion
  JABSve_d_TipsNum : Constant  OutDataTypeStr=uint8
  JABSve_d_Tips_1 : DataTypeConversion  OutDataTypeStr=UInt16
  System_Clock_convert : DataTypeConversion  OutDataTypeStr=uint8
  JABSve_d_Switching : Outport  OutDataTypeStr=UInt16
  JABSve_d_DecelReq : Outport  Port=2  OutDataTypeStr=T_M_Nm_Float32
  JABSve_d_AlertSign : Outport  Port=3  OutDataTypeStr=UInt16
  JABSve_d_SwitchStatus : Outport  Port=4  OutDataTypeStr=UInt16
  JABSve_d_FltStatus : Outport  Port=5  OutDataTypeStr=UInt16
  JABSve_d_AlertReq : Outport  Port=6  OutDataTypeStr=UInt16
  JABSve_d_HapticAlarm : Outport  Port=7  OutDataTypeStr=UInt16
  JABSve_d_Tips : Outport  Port=8  OutDataTypeStr=UInt16
  JABSve_d_DbPrefillReq : Outport  Port=9  OutDataTypeStr=UInt16
  JABSve_d_DbFunFARCSta : Outport  Port=10  OutDataTypeStr=UInt16
  JABSve_d_DbDecSetpoint : Outport  Port=11  OutDataTypeStr=T_M_Nm_Float32
  JABSve_d_DbMDDdecRequest : Outport  Port=12  OutDataTypeStr=UInt16
  JABSve_d_DbMDDdecType : Outport  Port=13  OutDataTypeStr=UInt16
  JABSve_d_DbHapticAlarm : Outport  Port=14  OutDataTypeStr=UInt16
  JABSve_d_DbSignalTStamp : Outport  Port=15  OutDataTypeStr=UInt16
  JABSve_d_DbAlertSign : Outport  Port=16  OutDataTypeStr=UInt16
  JABSve_d_DbSwitchStatus : Outport  Port=17  OutDataTypeStr=UInt16
  JABSve_d_DbFltStatus : Outport  Port=18  OutDataTypeStr=UInt16
  JABSve_d_DbAlertReq : Outport  Port=19  OutDataTypeStr=UInt16
  JABSve_d_DbTips : Outport  Port=20  OutDataTypeStr=UInt16
  wires:
  System_Clock/1 -> System_Clock_convert/1
  FDMMve_d_JaFcnConf/1 -> FDMMve_d_JaFcnConf_convert/1
  FDMMve_d_JaFcnConf_convert/1 -> FDMMve_d_JaFcnConf_1/1
  FDMMve_d_SignalTStamp/1 -> FDMMve_d_SignalTStamp_convert/1
  FDMMve_d_SignalTStamp_convert/1 -> FDMMve_d_SignalTStamp_1/1
  IMAPve_g_EPS_SW_Trq/1 -> IMAPve_g_EPS_SW_Trq_convert/1
  IMAPve_g_EPS_SW_Trq_convert/1 -> IMAPve_g_EPS_SW_Trq_1/1
  IMAPve_d_EPS_Error_State/1 -> IMAPve_d_EPS_Error_State_convert/1
  IMAPve_d_EPS_Error_State_convert/1 -> IMAPve_d_EPS_Error_State_1/1
  IMAPve_g_ESC_LatAcc/1 -> IMAPve_g_ESC_LatAcc_convert/1
  IMAPve_g_ESC_LatAcc_convert/1 -> IMAPve_g_ESC_LatAcc_1/1
  IMAPve_g_ESC_YawRate/1 -> IMAPve_g_ESC_YawRate_convert/1
  IMAPve_g_ESC_YawRate_convert/1 -> IMAPve_g_ESC_YawRate_1/1
  IMAPve_d_ESC_YawRate_Valid/1 -> IMAPve_d_ESC_YawRate_Valid_convert/1
  IMAPve_d_ESC_YawRate_Valid_convert/1 -> IMAPve_d_ESC_YawRate_Valid_1/1
  IMAPve_g_ESC_UnYawRate/1 -> IMAPve_g_ESC_UnYawRate_convert/1
  IMAPve_g_ESC_UnYawRate_convert/1 -> IMAPve_g_ESC_UnYawRate_1/1
  IMAPve_g_ESC_VehSpd/1 -> IMAPve_g_ESC_VehSpd_convert/1
  IMAPve_g_ESC_VehSpd_convert/1 -> IMAPve_g_ESC_VehSpd_1/1
  IMAPve_g_ESC_LonAcc/1 -> IMAPve_g_ESC_LonAcc_convert/1
  IMAPve_g_ESC_LonAcc_convert/1 -> IMAPve_g_ESC_LonAcc_1/1
  IMAPve_d_ESC_LonAcc_Valid/1 -> IMAPve_d_ESC_LonAcc_Valid_convert/1
  IMAPve_d_ESC_LonAcc_Valid_convert/1 -> IMAPve_d_ESC_LonAcc_Valid_1/1
  IMAPve_g_ESC_Brake_Press/1 -> IMAPve_g_ESC_Brake_Press_convert/1
  IMAPve_g_ESC_Brake_Press_convert/1 -> IMAPve_g_ESC_Brake_Press_1/1
  IMAPve_g_ESC_Static_Slope/1 -> IMAPve_g_ESC_Static_Slope_convert/1
  IMAPve_g_ESC_Static_Slope_convert/1 -> IMAPve_g_ESC_Static_Slope_1/1
  IMAPve_g_ESC_DySlope_Accuracy/1 -> IMAPve_g_ESC_DySlope_Accuracy_convert/1
  IMAPve_g_ESC_DySlope_Accuracy_convert/1 -> IMAPve_g_ESC_DySlope_Accuracy_1/1
  IMAPve_g_ESC_DySlope/1 -> IMAPve_g_ESC_DySlope_convert/1
  IMAPve_g_ESC_DySlope_convert/1 -> IMAPve_g_ESC_DySlope_1/1
  IMAPve_g_SW_Angle/1 -> IMAPve_g_SW_Angle_convert/1
  IMAPve_g_SW_Angle_convert/1 -> IMAPve_g_SW_Angle_1/1
  IMAPve_g_SW_Angle_Speed/1 -> IMAPve_g_SW_Angle_Speed_convert/1
  IMAPve_g_SW_Angle_Speed_convert/1 -> IMAPve_g_SW_Angle_Speed_1/1
  IMAPve_d_BCM_HazardLamp/1 -> IMAPve_d_BCM_HazardLamp_convert/1
  IMAPve_d_BCM_HazardLamp_convert/1 -> IMAPve_d_BCM_HazardLamp_1/1
  IMAPve_d_BCM_Left_Light/1 -> IMAPve_d_BCM_Left_Light_convert/1
  IMAPve_d_BCM_Left_Light_convert/1 -> IMAPve_d_BCM_Left_Light_1/1
  IMAPve_d_BCM_Right_Light/1 -> IMAPve_d_BCM_Right_Light_convert/1
  IMAPve_d_BCM_Right_Light_convert/1 -> IMAPve_d_BCM_Right_Light_1/1
  IMAPve_d_BCM_Opening_State/1 -> IMAPve_d_BCM_Opening_State_convert/1
  IMAPve_d_BCM_Opening_State_convert/1 -> IMAPve_d_BCM_Opening_State_1/1
  IMAPve_d_SCC_Left_SwitchSig/1 -> IMAPve_d_SCC_Left_SwitchSig_convert/1
  IMAPve_d_SCC_Left_SwitchSig_convert/1 -> IMAPve_d_SCC_Left_SwitchSig_1/1
  IMAPve_d_SCC_Right_SwitchSig/1 -> IMAPve_d_SCC_Right_SwitchSig_convert/1
  IMAPve_d_SCC_Right_SwitchSig_convert/1 -> IMAPve_d_SCC_Right_SwitchSig_1/1
  IMAPve_g_EMS_RealPedal/1 -> IMAPve_g_EMS_RealPedal_convert/1
  IMAPve_g_EMS_RealPedal_convert/1 -> IMAPve_g_EMS_RealPedal_1/1
  IMAPve_g_EMS_ACC_VirtualPedal/1 -> IMAPve_g_EMS_ACC_VirtualPedal_convert/1
  IMAPve_g_EMS_ACC_VirtualPedal_convert/1 -> IMAPve_g_EMS_ACC_VirtualPedal_1/1
  IMAPve_d_ESC_Veh_Standstill/1 -> IMAPve_d_ESC_Veh_Standstill_convert/1
  IMAPve_d_ESC_Veh_Standstill_convert/1 -> IMAPve_d_ESC_Veh_Standstill_1/1
  IMAPve_d_TCU_Actual_Gear/1 -> IMAPve_d_TCU_Actual_Gear_convert/1
  IMAPve_d_TCU_Actual_Gear_convert/1 -> IMAPve_d_TCU_Actual_Gear_1/1
  IMAPve_d_TCU_Target_Gear/1 -> IMAPve_d_TCU_Target_Gear_convert/1
  IMAPve_d_TCU_Target_Gear_convert/1 -> IMAPve_d_TCU_Target_Gear_1/1
  IMAPve_d_BCM_Ignition_State/1 -> IMAPve_d_BCM_Ignition_State_convert/1
  IMAPve_d_BCM_Ignition_State_convert/1 -> IMAPve_d_BCM_Ignition_State_1/1
  IMAPve_d_ACU_Driver_Belt/1 -> IMAPve_d_ACU_Driver_Belt_convert/1
  IMAPve_d_ACU_Driver_Belt_convert/1 -> IMAPve_d_ACU_Driver_Belt_1/1
  IMAPve_d_SWS_Fault_Code/1 -> IMAPve_d_SWS_Fault_Code_convert/1
  IMAPve_d_SWS_Fault_Code_convert/1 -> IMAPve_d_SWS_Fault_Code_1/1
  IMAPve_d_SWS_Failure_Status/1 -> IMAPve_d_SWS_Failure_Status_convert/1
  IMAPve_d_SWS_Failure_Status_convert/1 -> IMAPve_d_SWS_Failure_Status_1/1
  IMAPve_d_ESC_OFF/1 -> IMAPve_d_ESC_OFF_convert/1
  IMAPve_d_ESC_OFF_convert/1 -> IMAPve_d_ESC_OFF_1/1
  IMAPve_d_ESC_AlarmSig/1 -> IMAPve_d_ESC_AlarmSig_convert/1
  IMAPve_d_ESC_AlarmSig_convert/1 -> IMAPve_d_ESC_AlarmSig_1/1
  IMAPve_d_ESC_ESC_Active/1 -> IMAPve_d_ESC_ESC_Active_convert/1
  IMAPve_d_ESC_ESC_Active_convert/1 -> IMAPve_d_ESC_ESC_Active_1/1
  IMAPve_d_ESC_MSR_Active/1 -> IMAPve_d_ESC_MSR_Active_convert/1
  IMAPve_d_ESC_MSR_Active_convert/1 -> IMAPve_d_ESC_MSR_Active_1/1
  IMAPve_d_ESC_TCS_Active/1 -> IMAPve_d_ESC_TCS_Active_convert/1
  IMAPve_d_ESC_TCS_Active_convert/1 -> IMAPve_d_ESC_TCS_Active_1/1
  IMAPve_d_ESC_VehSpd_Valid/1 -> IMAPve_d_ESC_VehSpd_Valid_convert/1
  IMAPve_d_ESC_VehSpd_Valid_convert/1 -> IMAPve_d_ESC_VehSpd_Valid_1/1
  IMAPve_d_Brake_Pedal_Fault/1 -> IMAPve_d_Brake_Pedal_Fault_convert/1
  IMAPve_d_Brake_Pedal_Fault_convert/1 -> IMAPve_d_Brake_Pedal_Fault_1/1
  IMAPve_d_ESC_ABS_Active/1 -> IMAPve_d_ESC_ABS_Active_convert/1
  IMAPve_d_ESC_ABS_Active_convert/1 -> IMAPve_d_ESC_ABS_Active_1/1
  IMAPve_d_ESC_FL_WheelPulVal/1 -> IMAPve_d_ESC_FL_WheelPulVal_convert/1
  IMAPve_d_ESC_FL_WheelPulVal_convert/1 -> IMAPve_d_ESC_FL_WheelPulVal_1/1
  IMAPve_d_ESC_FR_WheelPulVal/1 -> IMAPve_d_ESC_FR_WheelPulVal_convert/1
  IMAPve_d_ESC_FR_WheelPulVal_convert/1 -> IMAPve_d_ESC_FR_WheelPulVal_1/1
  IMAPve_d_ESC_RL_WheelPulVal/1 -> IMAPve_d_ESC_RL_WheelPulVal_convert/1
  IMAPve_d_ESC_RL_WheelPulVal_convert/1 -> IMAPve_d_ESC_RL_WheelPulVal_1/1
  IMAPve_d_ESC_RR_WheelPulVal/1 -> IMAPve_d_ESC_RR_WheelPulVal_convert/1
  IMAPve_d_ESC_RR_WheelPulVal_convert/1 -> IMAPve_d_ESC_RR_WheelPulVal_1/1
  IMAPve_d_TCU_AT_Failure/1 -> IMAPve_d_TCU_AT_Failure_convert/1
  IMAPve_d_TCU_AT_Failure_convert/1 -> IMAPve_d_TCU_AT_Failure_1/1
  IMAPve_d_EMS_Engine_Status/1 -> IMAPve_d_EMS_Engine_Status_convert/1
  IMAPve_d_EMS_Engine_Status_convert/1 -> IMAPve_d_EMS_Engine_Status_1/1
  IMAPve_d_ESC_AEB_Status/1 -> IMAPve_d_ESC_AEB_Status_convert/1
  IMAPve_d_ESC_AEB_Status_convert/1 -> IMAPve_d_ESC_AEB_Status_1/1
  IMAPve_d_ESC_AEB_Available/1 -> IMAPve_d_ESC_AEB_Available_convert/1
  IMAPve_d_ESC_AEB_Available_convert/1 -> IMAPve_d_ESC_AEB_Available_1/1
  IMAPve_d_ESC_AEB_Active/1 -> IMAPve_d_ESC_AEB_Active_convert/1
  IMAPve_d_ESC_AEB_Active_convert/1 -> IMAPve_d_ESC_AEB_Active_1/1
  IMAPve_d_BCM_FrontWiper_State/1 -> IMAPve_d_BCM_FrontWiper_State_convert/1
  IMAPve_d_BCM_FrontWiper_State_convert/1 -> IMAPve_d_BCM_FrontWiper_State_1/1
  IMAPve_d_BCM_CHMSL_Status/1 -> IMAPve_d_BCM_CHMSL_Status_convert/1
  IMAPve_d_BCM_CHMSL_Status_convert/1 -> IMAPve_d_BCM_CHMSL_Status_1/1
  IMAPve_d_BCM_BrakeLamp_State/1 -> IMAPve_d_BCM_BrakeLamp_State_convert/1
  IMAPve_d_BCM_BrakeLamp_State_convert/1 -> IMAPve_d_BCM_BrakeLamp_State_1/1
  IMAPve_d_ACU_Passenger_Belt/1 -> IMAPve_d_ACU_Passenger_Belt_convert/1
  IMAPve_d_ACU_Passenger_Belt_convert/1 -> IMAPve_d_ACU_Passenger_Belt_1/1
  IMAPve_d_EMS_Brake_Pedal/1 -> IMAPve_d_EMS_Brake_Pedal_convert/1
  IMAPve_d_EMS_Brake_Pedal_convert/1 -> IMAPve_d_EMS_Brake_Pedal_1/1
  IMAPve_d_EPB_Status/1 -> IMAPve_d_EPB_Status_convert/1
  IMAPve_d_EPB_Status_convert/1 -> IMAPve_d_EPB_Status_1/1
  IMAPve_d_ESC_Drive_Direction/1 -> IMAPve_d_ESC_Drive_Direction_convert/1
  IMAPve_d_ESC_Drive_Direction_convert/1 -> IMAPve_d_ESC_Drive_Direction_1/1
  IMAPve_d_ESC_Hold_State/1 -> IMAPve_d_ESC_Hold_State_convert/1
  IMAPve_d_ESC_Hold_State_convert/1 -> IMAPve_d_ESC_Hold_State_1/1
  IMAPve_d_Radar_State/1 -> IMAPve_d_Radar_State_convert/1
  IMAPve_d_Radar_State_convert/1 -> IMAPve_d_Radar_State_1/1
  IMAPve_d_Signal_Time_Stamp/1 -> IMAPve_d_Signal_Time_Stamp_convert/1
  IMAPve_d_Signal_Time_Stamp_convert/1 -> IMAPve_d_Signal_Time_Stamp_1/1
  IMAPve_d_Sensor_Status/1 -> IMAPve_d_Sensor_Status_convert/1
  IMAPve_d_Sensor_Status_convert/1 -> IMAPve_d_Sensor_Status_1/1
  IMAPve_d_LF_Radar_Status/1 -> IMAPve_d_LF_Radar_Status_convert/1
  IMAPve_d_LF_Radar_Status_convert/1 -> IMAPve_d_LF_Radar_Status_1/1
  IMAPve_d_RF_Radar_Status/1 -> IMAPve_d_RF_Radar_Status_convert/1
  IMAPve_d_RF_Radar_Status_convert/1 -> IMAPve_d_RF_Radar_Status_1/1
  IMAPve_d_LR_Radar_Status/1 -> IMAPve_d_LR_Radar_Status_convert/1
  IMAPve_d_LR_Radar_Status_convert/1 -> IMAPve_d_LR_Radar_Status_1/1
  IMAPve_d_RR_Radar_Status/1 -> IMAPve_d_RR_Radar_Status_convert/1
  IMAPve_d_RR_Radar_Status_convert/1 -> IMAPve_d_RR_Radar_Status_1/1
  IMAPve_d_Fusion_Status/1 -> IMAPve_d_Fusion_Status_convert/1
  IMAPve_d_Fusion_Status_convert/1 -> IMAPve_d_Fusion_Status_1/1
  IMAPve_g_Fusion_Time_Stamp/1 -> IMAPve_g_Fusion_Time_Stamp_convert/1
  IMAPve_g_Fusion_Time_Stamp_convert/1 -> IMAPve_g_Fusion_Time_Stamp_1/1
  IMAPve_d_obj_Num/1 -> IMAPve_d_obj_Num_convert/1
  IMAPve_d_obj_Num_convert/1 -> IMAPve_d_obj_Num_1/1
  IMAPva_d_obj_id/1 -> IMAPva_d_obj_id_convert/1
  IMAPva_d_obj_id_convert/1 -> IMAPva_d_obj_id_1/1
  IMAPva_g_obj_pos_x/1 -> IMAPva_g_obj_pos_x_convert/1
  IMAPva_g_obj_pos_x_convert/1 -> IMAPva_g_obj_pos_x_1/1
  IMAPva_g_obj_pos_y/1 -> IMAPva_g_obj_pos_y_convert/1
  IMAPva_g_obj_pos_y_convert/1 -> IMAPva_g_obj_pos_y_1/1
  IMAPva_g_obj_vel_x/1 -> IMAPva_g_obj_vel_x_convert/1
  IMAPva_g_obj_vel_x_convert/1 -> IMAPva_g_obj_vel_x_1/1
  IMAPva_g_obj_vel_y/1 -> IMAPva_g_obj_vel_y_convert/1
  IMAPva_g_obj_vel_y_convert/1 -> IMAPva_g_obj_vel_y_1/1
  IMAPva_g_obj_acc_x/1 -> IMAPva_g_obj_acc_x_convert/1
  IMAPva_g_obj_acc_x_convert/1 -> IMAPva_g_obj_acc_x_1/1
  IMAPva_g_obj_acc_y/1 -> IMAPva_g_obj_acc_y_convert/1
  IMAPva_g_obj_acc_y_convert/1 -> IMAPva_g_obj_acc_y_1/1
  IMAPva_g_obj_pos_var_x/1 -> IMAPva_g_obj_pos_var_x_convert/1
  IMAPva_g_obj_pos_var_x_convert/1 -> IMAPva_g_obj_pos_var_x_1/1
  IMAPva_g_obj_pos_var_y/1 -> IMAPva_g_obj_pos_var_y_convert/1
  IMAPva_g_obj_pos_var_y_convert/1 -> IMAPva_g_obj_pos_var_y_1/1
  IMAPva_g_obj_pos_var_xy/1 -> IMAPva_g_obj_pos_var_xy_convert/1
  IMAPva_g_obj_pos_var_xy_convert/1 -> IMAPva_g_obj_pos_var_xy_1/1
  IMAPva_g_obj_vel_var_x/1 -> IMAPva_g_obj_vel_var_x_convert/1
  IMAPva_g_obj_vel_var_x_convert/1 -> IMAPva_g_obj_vel_var_x_1/1
  IMAPva_g_obj_vel_var_y/1 -> IMAPva_g_obj_vel_var_y_convert/1
  IMAPva_g_obj_vel_var_y_convert/1 -> IMAPva_g_obj_vel_var_y_1/1
  IMAPva_g_obj_vel_var_xy/1 -> IMAPva_g_obj_vel_var_xy_convert/1
  IMAPva_g_obj_vel_var_xy_convert/1 -> IMAPva_g_obj_vel_var_xy_1/1
  IMAPva_g_obj_width/1 -> IMAPva_g_obj_width_convert/1
  IMAPva_g_obj_width_convert/1 -> IMAPva_g_obj_width_1/1
  IMAPva_g_obj_length/1 -> IMAPva_g_obj_length_convert/1
  IMAPva_g_obj_length_convert/1 -> IMAPva_g_obj_length_1/1
  IMAPva_d_obj_fusion_type/1 -> IMAPva_d_obj_fusion_type_convert/1
  IMAPva_d_obj_fusion_type_convert/1 -> IMAPva_d_obj_fusion_type_1/1
  IMAPva_d_obj_class/1 -> IMAPva_d_obj_class_convert/1
  IMAPva_d_obj_class_convert/1 -> IMAPva_d_obj_class_1/1
  IMAPva_d_obj_lane/1 -> IMAPva_d_obj_lane_convert/1
  IMAPva_d_obj_lane_convert/1 -> IMAPva_d_obj_lane_1/1
  IMAPva_d_obj_status/1 -> IMAPva_d_obj_status_convert/1
  IMAPva_d_obj_status_convert/1 -> IMAPva_d_obj_status_1/1
  IMAPva_d_obj_cam_asso_id/1 -> IMAPva_d_obj_cam_asso_id_convert/1
  IMAPva_d_obj_cam_asso_id_convert/1 -> IMAPva_d_obj_cam_asso_id_1/1
  IMAPva_g_obj_con/1 -> IMAPva_g_obj_con_convert/1
  IMAPva_g_obj_con_convert/1 -> IMAPva_g_obj_con_1/1
  IMAPva_g_obj_age/1 -> IMAPva_g_obj_age_convert/1
  IMAPva_g_obj_age_convert/1 -> IMAPva_g_obj_age_1/1
  IMAPva_d_obj_TurnLight/1 -> IMAPva_d_obj_TurnLight_convert/1
  IMAPva_d_obj_TurnLight_convert/1 -> IMAPva_d_obj_TurnLight_1/1
  IMAPva_d_obj_BrakeLight/1 -> IMAPva_d_obj_BrakeLight_convert/1
  IMAPva_d_obj_BrakeLight_convert/1 -> IMAPva_d_obj_BrakeLight_1/1
  IMAPva_d_obj_MotionStatus/1 -> IMAPva_d_obj_MotionStatus_convert/1
  IMAPva_d_obj_MotionStatus_convert/1 -> IMAPva_d_obj_MotionStatus_1/1
  IMAPva_d_obj_AEB/1 -> IMAPva_d_obj_AEB_convert/1
  IMAPva_d_obj_AEB_convert/1 -> IMAPva_d_obj_AEB_1/1
  IMAPva_d_obj_ESA/1 -> IMAPva_d_obj_ESA_convert/1
  IMAPva_d_obj_ESA_convert/1 -> IMAPva_d_obj_ESA_1/1
  IMAPva_d_obj_JA/1 -> IMAPva_d_obj_JA_convert/1
  IMAPva_d_obj_JA_convert/1 -> IMAPva_d_obj_JA_1/1
  IMAPve_d_Lane_Valid/1 -> IMAPve_d_Lane_Valid_convert/1
  IMAPve_d_Lane_Valid_convert/1 -> IMAPve_d_Lane_Valid_1/1
  IMAPve_d_Road_Type/1 -> IMAPve_d_Road_Type_convert/1
  IMAPve_d_Road_Type_convert/1 -> IMAPve_d_Road_Type_1/1
  IMAPve_d_ConsArea/1 -> IMAPve_d_ConsArea_convert/1
  IMAPve_d_ConsArea_convert/1 -> IMAPve_d_ConsArea_1/1
  IMAPve_g_L0_C0/1 -> IMAPve_g_L0_C0_convert/1
  IMAPve_g_L0_C0_convert/1 -> IMAPve_g_L0_C0_1/1
  IMAPve_g_L0_C1/1 -> IMAPve_g_L0_C1_convert/1
  IMAPve_g_L0_C1_convert/1 -> IMAPve_g_L0_C1_1/1
  IMAPve_g_L0_C2/1 -> IMAPve_g_L0_C2_convert/1
  IMAPve_g_L0_C2_convert/1 -> IMAPve_g_L0_C2_1/1
  IMAPve_g_L0_C3/1 -> IMAPve_g_L0_C3_convert/1
  IMAPve_g_L0_C3_convert/1 -> IMAPve_g_L0_C3_1/1
  IMAPve_g_L0_VR/1 -> IMAPve_g_L0_VR_convert/1
  IMAPve_g_L0_VR_convert/1 -> IMAPve_g_L0_VR_1/1
  IMAPve_d_L0_Q/1 -> IMAPve_d_L0_Q_convert/1
  IMAPve_d_L0_Q_convert/1 -> IMAPve_d_L0_Q_1/1
  IMAPve_d_L0_Type/1 -> IMAPve_d_L0_Type_convert/1
  IMAPve_d_L0_Type_convert/1 -> IMAPve_d_L0_Type_1/1
  IMAPve_g_L0_Confidence/1 -> IMAPve_g_L0_Confidence_convert/1
  IMAPve_g_L0_Confidence_convert/1 -> IMAPve_g_L0_Confidence_1/1
  IMAPve_g_L0_W/1 -> IMAPve_g_L0_W_convert/1
  IMAPve_g_L0_W_convert/1 -> IMAPve_g_L0_W_1/1
  IMAPve_g_L0_TLC/1 -> IMAPve_g_L0_TLC_convert/1
  IMAPve_g_L0_TLC_convert/1 -> IMAPve_g_L0_TLC_1/1
  IMAPve_d_L0_LC/1 -> IMAPve_d_L0_LC_convert/1
  IMAPve_d_L0_LC_convert/1 -> IMAPve_d_L0_LC_1/1
  IMAPve_g_R0_C0/1 -> IMAPve_g_R0_C0_convert/1
  IMAPve_g_R0_C0_convert/1 -> IMAPve_g_R0_C0_1/1
  IMAPve_g_R0_C1/1 -> IMAPve_g_R0_C1_convert/1
  IMAPve_g_R0_C1_convert/1 -> IMAPve_g_R0_C1_1/1
  IMAPve_g_R0_C2/1 -> IMAPve_g_R0_C2_convert/1
  IMAPve_g_R0_C2_convert/1 -> IMAPve_g_R0_C2_1/1
  IMAPve_g_R0_C3/1 -> IMAPve_g_R0_C3_convert/1
  IMAPve_g_R0_C3_convert/1 -> IMAPve_g_R0_C3_1/1
  IMAPve_g_R0_VR/1 -> IMAPve_g_R0_VR_convert/1
  IMAPve_g_R0_VR_convert/1 -> IMAPve_g_R0_VR_1/1
  IMAPve_d_R0_Q/1 -> IMAPve_d_R0_Q_convert/1
  IMAPve_d_R0_Q_convert/1 -> IMAPve_d_R0_Q_1/1
  IMAPve_d_R0_Type/1 -> IMAPve_d_R0_Type_convert/1
  IMAPve_d_R0_Type_convert/1 -> IMAPve_d_R0_Type_1/1
  IMAPve_g_R0_Confidence/1 -> IMAPve_g_R0_Confidence_convert/1
  IMAPve_g_R0_Confidence_convert/1 -> IMAPve_g_R0_Confidence_1/1
  IMAPve_g_R0_W/1 -> IMAPve_g_R0_W_convert/1
  IMAPve_g_R0_W_convert/1 -> IMAPve_g_R0_W_1/1
  IMAPve_g_R0_TLC/1 -> IMAPve_g_R0_TLC_convert/1
  IMAPve_g_R0_TLC_convert/1 -> IMAPve_g_R0_TLC_1/1
  IMAPve_d_Sign_ISA_Value/1 -> IMAPve_d_Sign_ISA_Value_convert/1
  IMAPve_d_Sign_ISA_Value_convert/1 -> IMAPve_d_Sign_ISA_Value_1/1
  IMAPve_d_TSR_Sign_Type/1 -> IMAPve_d_TSR_Sign_Type_convert/1
  IMAPve_d_TSR_Sign_Type_convert/1 -> IMAPve_d_TSR_Sign_Type_1/1
  IMAPve_d_Camera_Signal_Fault/1 -> IMAPve_d_Camera_Signal_Fault_convert/1
  IMAPve_d_Camera_Signal_Fault_convert/1 -> IMAPve_d_Camera_Signal_Fault_1/1
  IMAPve_d_Radar_Status/1 -> IMAPve_d_Radar_Status_convert/1
  IMAPve_d_Radar_Status_convert/1 -> IMAPve_d_Radar_Status_1/1
  IMAPve_d_Camera_Status/1 -> IMAPve_d_Camera_Status_convert/1
  IMAPve_d_Camera_Status_convert/1 -> IMAPve_d_Camera_Status_1/1
  System_Clock_convert/1 -> JABSve_d_Switching_1/1
  JABSve_d_Switching_1/1 -> JABSve_d_Switching/1
  JABSve_d_DecelReqNum/1 -> JABSve_d_DecelReq_1/1
  JABSve_d_DecelReq_1/1 -> JABSve_d_DecelReq/1
  JABSve_d_AlertSignNum/1 -> JABSve_d_AlertSign_1/1
  JABSve_d_AlertSign_1/1 -> JABSve_d_AlertSign/1
  JABSve_d_SwitchStatusNum/1 -> JABSve_d_SwitchStatus_1/1
  JABSve_d_SwitchStatus_1/1 -> JABSve_d_SwitchStatus/1
  JABSve_d_FltStatusNum/1 -> JABSve_d_FltStatus_1/1
  JABSve_d_FltStatus_1/1 -> JABSve_d_FltStatus/1
  JABSve_d_AlertReqNum/1 -> JABSve_d_AlertReq_1/1
  JABSve_d_AlertReq_1/1 -> JABSve_d_AlertReq/1
  JABSve_d_HapticAlarmNum/1 -> JABSve_d_HapticAlarm_1/1
  JABSve_d_HapticAlarm_1/1 -> JABSve_d_HapticAlarm/1
  JABSve_d_TipsNum/1 -> JABSve_d_Tips_1/1
  JABSve_d_Tips_1/1 -> JABSve_d_Tips/1
  JABSve_d_DbPrefillReqNum/1 -> JABSve_d_DbPrefillReq_1/1
  JABSve_d_DbPrefillReq_1/1 -> JABSve_d_DbPrefillReq/1
  JABSve_d_DbFunFARCStaNum/1 -> JABSve_d_DbFunFARCSta_1/1
  JABSve_d_DbFunFARCSta_1/1 -> JABSve_d_DbFunFARCSta/1
  JABSve_d_DbDecSetpointNum/1 -> JABSve_d_DbDecSetpoint_1/1
  JABSve_d_DbDecSetpoint_1/1 -> JABSve_d_DbDecSetpoint/1
  JABSve_d_DbMDDdecRequestNum/1 -> JABSve_d_DbMDDdecRequest_1/1
  JABSve_d_DbMDDdecRequest_1/1 -> JABSve_d_DbMDDdecRequest/1
  JABSve_d_DbMDDdecTypeNum/1 -> JABSve_d_DbMDDdecType_1/1
  JABSve_d_DbMDDdecType_1/1 -> JABSve_d_DbMDDdecType/1
  JABSve_d_DbHapticAlarmNum/1 -> JABSve_d_DbHapticAlarm_1/1
  JABSve_d_DbHapticAlarm_1/1 -> JABSve_d_DbHapticAlarm/1
  JABSve_d_DbSignalTStampNum/1 -> JABSve_d_DbSignalTStamp_1/1
  JABSve_d_DbSignalTStamp_1/1 -> JABSve_d_DbSignalTStamp/1
  JABSve_d_DbAlertSignNum/1 -> JABSve_d_DbAlertSign_1/1
  JABSve_d_DbAlertSign_1/1 -> JABSve_d_DbAlertSign/1
  JABSve_d_DbSwitchStatusNum/1 -> JABSve_d_DbSwitchStatus_1/1
  JABSve_d_DbSwitchStatus_1/1 -> JABSve_d_DbSwitchStatus/1
  JABSve_d_DbFltStatusNum/1 -> JABSve_d_DbFltStatus_1/1
  JABSve_d_DbFltStatus_1/1 -> JABSve_d_DbFltStatus/1
  JABSve_d_DbAlertReqNum/1 -> JABSve_d_DbAlertReq_1/1
  JABSve_d_DbAlertReq_1/1 -> JABSve_d_DbAlertReq/1
  JABSve_d_DbTipsNum/1 -> JABSve_d_DbTips_1/1
  JABSve_d_DbTips_1/1 -> JABSve_d_DbTips/1
